simulink model "MicrostickII_ExternalMode"  (R2017b)
settings: Solver=FixedStepDiscrete  StartTime=0.0  StopTime=inf  FixedStep=0.01  RelTol=1e-3
undefined symbols (not defined in the file): A4, B0, B10, B11, B12, Max, MaxPer, ms, P20, P32, P42, P43, Pin, Resol, s, us
libraries: MCHP_Blockset x10
settings Model: SimulationMode=external  ExtModeTrigDuration=1  Creator=M17129  LastModifiedBy=m17129
settings OptimizationCC: PassReuseOutputArgsAs=Individual arguments
settings DebuggingCC: ParameterTunabilityLossMsg=error
settings HardwareCC: ProdBitPerInt=16  ProdBitPerPointer=16  ProdBitPerSizeT=16  ProdBitPerPtrDiffT=16  ProdLargestAtomicInteger=Integer  ProdLargestAtomicFloat=None  ProdWordSize=16  ProdHWDeviceType=Generic->Custom
settings ModelReferenceCC: ModelReferenceNumInstancesAllowed=Single
settings SFSimCC: MATLABDynamicMemAlloc=off
settings RTWCC: SystemTargetFile=MCHP_dsPIC_stf.tlc  TemplateMakefile=MCHP_dsPIC.tmf  Description=Microchip Embedded Target PIC24 dsPIC30 dsPIC33 (real-time)  GenerateReport=on  IncludeHyperlinkInReport=on  LaunchReport=on  CodeExecutionProfiling=on  CodeProfilingInstrumentation=on  GenerateTraceInfo=on  GenerateTraceReport=on  GenerateTraceReportSl=on  GenerateTraceReportSf=on  GenerateTraceReportEml=on  GenerateWebview=on  GenerateCodeMetricsReport=on  GenerateCodeReplacementReport=on
settings CodeAppCC: ForceParamTrailComments=on  IgnoreCustomStorageClasses=off  MaxIdLength=255  OperatorAnnotations=on  SimulinkDataObjDesc=on  SFDataObjDesc=on  InsertBlockDesc=on
settings STFCustomTargetCC: TargetLibSuffix=_lib.a  CodeReplacementLibrary=Microchip® Code Replacement Library for dsPIC  MultiwordLength=256  IncludeMdlTerminateFcn=off  CombineOutputUpdateFcns=on  CombineSignalStateStructs=on  ERTCustomFileBanners=on  SupportContinuousTime=off  RemoveResetFunc=on  MATLABClassNameForMDSCustomization=Simulink.SoftwareTarget.ERTCustomization  GRTInterface=off  SystemTargetFile=MCHP_dsPIC_stf.tlc
settings ERTTargetCC: TargetLibSuffix=_lib.a  CodeReplacementLibrary=Microchip® Code Replacement Library for dsPIC  ParMdlRefBuildCompliant=off  CompOptLevelCompliant=off  ConcurrentExecutionCompliant=off  IncludeMdlTerminateFcn=off  CombineSignalStateStructs=on  SupportNonInlinedSFcns=on  ModelStepFunctionPrototypeControlCompliant=off  CPPClassGenCompliant=off  UseToolchainInfoCompliant=off  ExtMode=on  ExtModeStaticAlloc=on  ExtModeStaticAllocSize=9000  ExtModeMexFile=ext_serial_win32_comm_no_acks  ExtModeMexArgs=1 5 460800  ERTSrcFileBannerTemplate=MCHP_dsPIC_code_template.cgt  ERTHdrFileBannerTemplate=MCHP_dsPIC_code_template.cgt  ERTDataSrcFileTemplate=MCHP_dsPIC_code_template.cgt  ERTDataHdrFileTemplate=MCHP_dsPIC_code_template.cgt  ERTCustomFileTemplate=MCHP_main.tlc

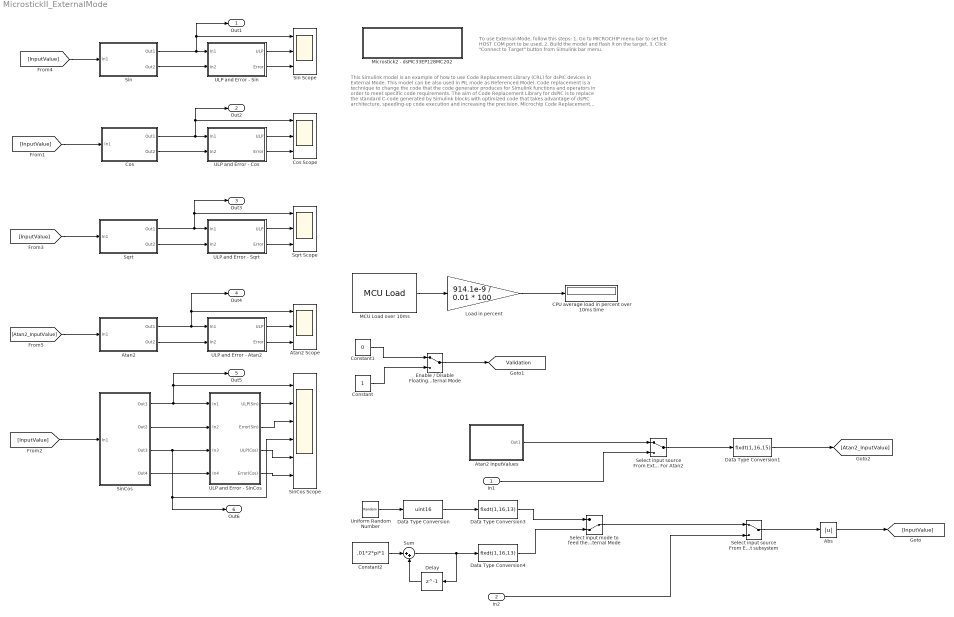
== system MicrostickII_ExternalMode ==
  note: This Simulink model is an example of how to use Code Replacement Library (CRL) for dsPIC devices in External Mode. This model can be also used in PIL mode as Referenced Model.
      |
      | Code replacement is a technique to change the code that the code generator produces for Simulink functions and operators
      | in order to meet specific code requirements. The aim of Code Replacement Library for dsPIC is to replace the standard C-code generated
      | by Simulink blocks with optimized code that takes advantage of dsPIC architecture, speeding-up code execution and increasing the precision.
      |
      | Microchip Code Replacement Library for dsPIC provides support for:
      | - Fixed-Point Matrix Multiplication operations
      | - Fixed-Point Atan2
      | - Fixed-Point Sqrt and Sqrt32
      | - Fixed-Point Sin
      | - Fixed-Point Cos
      | - Fixed-Point SinCos
      | - Abs (absolute value)
      | - Addition and Subtraction with Saturation
      | - Saturation and Cast operations
      |
      | The user can enable Code Replacement Library in two easy steps:
      | 1. Open Configuration Parameters of the Simulink Model
      | 2. From Code Generation --> Interface pane select "Microchip® Code Replacement Library for dsPIC".
      |
      | *You can check which blocks triggered the code replacement by inspecting Code Replacement Report displayed at the end of the build process.
      | *Since this model runs in External Mode you can change the values of tunable parameters (ex. input values for trigonometric functions).
  note: To use External-Mode, follow this steps:
      | 1. Go to MICROCHIP menu bar to set the HOST COM port to be used.
      | 2. Build the model and flash it on the target.
      | 3. Click "Connect to Target" button from Simulink bar menu.
  In1 : Inport  PortDimensions=2
  In2 : Inport  Port=2
  Abs : Abs
  Atan2 : Subsystem
  Atan2 InputValues : Subsystem
  Atan2 Scope : Scope  NumInputPorts=3
  CPU average load in percent over 10ms time : Display
  Constant : Constant  OutDataTypeStr=uint16
  Constant1 : Constant  Value=0  OutDataTypeStr=uint16
  Constant2 : Constant  Value=.01*2*pi*1  OutDataTypeStr=fixdt(1,16,2*pi/65536,0)  SampleTime=.01
  Cos : Subsystem
  Cos Scope : Scope  NumInputPorts=3
  Data Type Conversion : DataTypeConversion  OutDataTypeStr=uint16  ConvertRealWorld=Stored Integer (SI)
  Data Type Conversion1 : DataTypeConversion  OutDataTypeStr=fixdt(1,16,15)  ConvertRealWorld=Stored Integer (SI)
  Data Type Conversion3 : DataTypeConversion  OutDataTypeStr=fixdt(1,16,13)  ConvertRealWorld=Stored Integer (SI)
  Data Type Conversion4 : DataTypeConversion  OutDataTypeStr=fixdt(1,16,13)
  Delay : Delay  DelayLength=1  InitialCondition=0
  Enable / Disable Floating-Point Reference Output *Modifiable in External Mode : ManualSwitch
  Load in percent : Gain  Gain=914.1e-9 / 0.01 * 100  ParamDataTypeStr=Inherit: Inherit from 'Gain'  OutMin=[0]  OutMax=[20]  OutDataTypeStr=single
  MCU Load over 10ms : MCHP_Blockset/Profiling/MCU Load  MCULoadPin=Dynamic Options  MCULoadPin_TXT=None  MCULoadMeasure=on  TIMER_Resolution=Dynamic Options  TIMER_Resolution_TXT="Resol: 0.9143(us)  -  Max: 59.9(ms)"  MCHP_TIMER_REQUEST={MCU_Load}{MCU_Load}21:5:0:0:[]:4194304;  MCHP_TIMER_RESULT=[2 65535 ]  MCHP_MASTERLINK=MicrostickII_ExternalMode/Microstick2 - dsPIC33EP128MC202/Microchip Master  MCHP_COMPILED_INFO="CompiledSampleTime= [0.010000000000000000208   0 ];CompiledInportDataTypes=[ ];CompiledInportDataWidth=[];"  Info="Timer 2:  Resol: 914.0898379(ns)  -  Max: 59.9058(ms)"  SampleTime=0.01
      settings: SourceProductName=MPLAB® Device Blocks for Simulink®
  Microstick2 - dsPIC33EP128MC202 : Subsystem
  Select input mode to feed the functions under test *Modifiable in External Mode : ManualSwitch  CurrentSetting=0
  Select input source From External (input port) / From Current subsystem : ManualSwitch
  Select input source From External (input port) / From Current subsystem For Atan2 : ManualSwitch
  Sin : Subsystem
  Sin Scope : Scope  NumInputPorts=3
  SinCos : Subsystem
  SinCos Scope : Scope  NumInputPorts=6
  Sqrt : Subsystem
  "Sqrt Scope " : Scope  NumInputPorts=3
  Sum : Sum  Inputs=|++  OutDataTypeStr=Inherit: Same as first input
  ULP and Error - Atan2 : Subsystem
  ULP and Error - Cos : Subsystem
  ULP and Error - Sin : Subsystem
  ULP and Error - SinCos : Subsystem
  ULP and Error - Sqrt : Subsystem
  Uniform Random Number : UniformRandomNumber  Minimum=0  Maximum=2^16-1  SampleTime=.01
  Out1 : Outport
  Out2 : Outport  Port=2
  Out3 : Outport  Port=3
  Out4 : Outport  Port=4
  Out5 : Outport  Port=5
  Out6 : Outport  Port=6
  tag scope: Validation=global
  wires:
  [InputValue] -> Sin/1(In1)
  [InputValue] -> Cos/1(In1)
  Select input source From External (input port) / From Current subsystem/1 -> Abs/1
  In2/1 -> Select input source From External (input port) / From Current subsystem/2
  Data Type Conversion3/1 -> Select input mode to feed the functions under test *Modifiable in External Mode/1
  ULP and Error - Sqrt/2(Error) -> "Sqrt Scope "/3
  Cos/1(Out1) -> Cos Scope/1, Out2/1, ULP and Error - Cos/1(In1)
  SinCos/1(Out1) -> Out5/1, SinCos Scope/1, ULP and Error - SinCos/1(In1)
  Cos/2(Out2) -> ULP and Error - Cos/2(In2)
  Constant1/1 -> Enable / Disable Floating-Point Reference Output *Modifiable in External Mode/1
  SinCos/4(Out4) -> ULP and Error - SinCos/4(In4)
  Atan2/1(Out1) -> Atan2 Scope/1, Out4/1, ULP and Error - Atan2/1(In1)
  ULP and Error - Cos/2(Error) -> Cos Scope/3
  ULP and Error - SinCos/3(ULP(Cos)) -> SinCos Scope/5
  ULP and Error - Atan2/1(ULP) -> Atan2 Scope/2
  Delay/1 -> Sum/2
  ULP and Error - Sqrt/1(ULP) -> "Sqrt Scope "/2
  Sqrt/1(Out1) -> "Sqrt Scope "/1, Out3/1, ULP and Error - Sqrt/1(In1)
  Data Type Conversion4/1 -> Select input mode to feed the functions under test *Modifiable in External Mode/2
  Data Type Conversion1/1 -> [Atan2_InputValue]
  SinCos/3(Out3) -> SinCos Scope/4, Out6/1, ULP and Error - SinCos/3(In3)
  ULP and Error - SinCos/4(Error(Cos)) -> SinCos Scope/6
  Sin/2(Out2) -> ULP and Error - Sin/2(In2)
  ULP and Error - Atan2/2(Error) -> Atan2 Scope/3
  ULP and Error - Cos/1(ULP) -> Cos Scope/2
  Data Type Conversion/1 -> Data Type Conversion3/1
  Sqrt/2(Out2) -> ULP and Error - Sqrt/2(In2)
  SinCos/2(Out2) -> ULP and Error - SinCos/2(In2)
  ULP and Error - Sin/1(ULP) -> Sin Scope/2
  MCU Load over 10ms/1 -> Load in percent/1
  Constant2/1 -> Sum/1
  Atan2/2(Out2) -> ULP and Error - Atan2/2(In2)
  Sum/1 -> Data Type Conversion4/1, Delay/1
  Sin/1(Out1) -> Out1/1, Sin Scope/1, ULP and Error - Sin/1(In1)
  [InputValue] -> Sqrt/1(In1)
  Uniform Random Number/1 -> Data Type Conversion/1
  ULP and Error - SinCos/1(ULP(Sin)) -> SinCos Scope/2
  Enable / Disable Floating-Point Reference Output *Modifiable in External Mode/1 -> [Validation]
  Constant/1 -> Enable / Disable Floating-Point Reference Output *Modifiable in External Mode/2
  ULP and Error - Sin/2(Error) -> Sin Scope/3
  In1/1 -> Select input source From External (input port) / From Current subsystem For Atan2/2
  [InputValue] -> SinCos/1(In1)
  Abs/1 -> [InputValue]
  Select input mode to feed the functions under test *Modifiable in External Mode/1 -> Select input source From External (input port) / From Current subsystem/1
  Select input source From External (input port) / From Current subsystem For Atan2/1 -> Data Type Conversion1/1
  [Atan2_InputValue] -> Atan2/1(In1)
  Atan2 InputValues/1(Out1) -> Select input source From External (input port) / From Current subsystem For Atan2/1
  ULP and Error - SinCos/2(Error(Sin)) -> SinCos Scope/3
  Load in percent/1 -> CPU average load in percent over 10ms time/1

== system MicrostickII_ExternalMode/Atan2 ==
  In1 : Inport
  Atan2 Q15 : Subsystem
  Double Atan2 - Reference : Subsystem  TreatAsAtomicUnit=on
  Out1 : Outport
  Out2 : Outport  Port=2
  wires:
  In1/1 -> Atan2 Q15/1(In1), Double Atan2 - Reference/1(In1)
  Double Atan2 - Reference/1(Simulink_Out_Q1.15) -> Out2/1
  Atan2 Q15/1(Out1) -> Out1/1
  [Validation] -> Double Atan2 - Reference/Enable

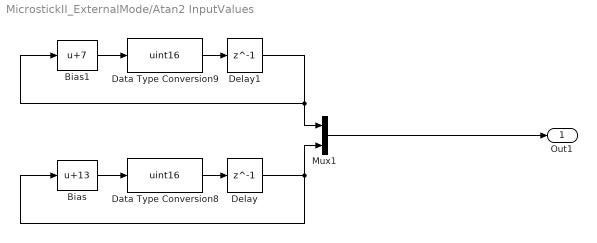
== system MicrostickII_ExternalMode/Atan2 InputValues ==
  Bias : Bias  Bias=13
  Bias1 : Bias  Bias=7
  Data Type Conversion8 : DataTypeConversion  OutDataTypeStr=uint16  ConvertRealWorld=Stored Integer (SI)
  Data Type Conversion9 : DataTypeConversion  OutDataTypeStr=uint16  ConvertRealWorld=Stored Integer (SI)
  Delay : Delay  DelayLength=1  InitialCondition=0
  Delay1 : Delay  DelayLength=1  InitialCondition=0
  Mux1 : Mux  Inputs=2
  Out1 : Outport
  wires:
  Delay/1 -> Bias/1, Mux1/2
  Data Type Conversion8/1 -> Delay/1
  Delay1/1 -> Mux1/1, Bias1/1
  Bias1/1 -> Data Type Conversion9/1
  Data Type Conversion9/1 -> Delay1/1
  Mux1/1 -> Out1/1
  Bias/1 -> Data Type Conversion8/1

== system MicrostickII_ExternalMode/Cos ==
  In1 : Inport
  Cos Double - Reference : Subsystem
  Cos Q15 : Subsystem
  Out1 : Outport
  Out2 : Outport  Port=2
  wires:
  In1/1 -> Cos Q15/1(In2), Cos Double - Reference/1(In1)
  Cos Double - Reference/1(Out1) -> Out2/1
  Cos Q15/1(Cos_Out1) -> Out1/1
  [Validation] -> Cos Double - Reference/Enable

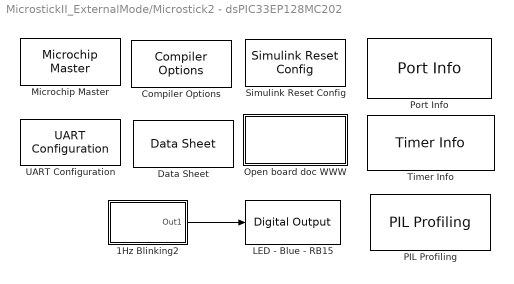
== system MicrostickII_ExternalMode/Microstick2 - dsPIC33EP128MC202 ==
  1Hz Blinking2 : Subsystem
  Compiler Options : MCHP_Blockset/System Configuration/Compiler Options  Priority=1  LATEST_CMPLR=on  COMP_LIST=Dynamic Options  COMP_LIST_TXT=xc16 - v1.33  USE_64BIT_DOUBLE=off  MCHP_MULTITHREAD_COMPILATION=on  UseCustom_LinkerScript=off  MCHP_MASTERLINK=MicrostickII_ExternalMode/Microstick2 - dsPIC33EP128MC202/Microchip Master  OPTIMIZATION_LEVEL=3  MPLAB_LINKLIB=default  MPLAB_LINKLIB1=default  UNROLL_LOOPS=on  OMIT_FRAME_POINTER=off  PROCEDURAL_ABSTRACTION=off  MCONST=in data memory  MDATA=Use only memory below address 8192 (faster)  MSCALAR=Use only memory below address 8192 (faster)  MCODE=is less than 32768 (faster)  HEAP_SIZE=0  OMF=elf  DEBUG_INFO=off  AssemblyListing=off  ProduceHexOutput=on
      settings: SourceProductName=MPLAB® Device Blocks for Simulink®
  Data Sheet : MCHP_Blockset/System Info/Data Sheet  DOC_Type=datasheet  DOC_MCHP_Id=33FJ64MC802  DOC_FileLastCheckTime=[0 0 0 0 0 0]  cpy_MCHP_Id=33EP128MC202  MCHP_MASTERLINK=MicrostickII_ExternalMode/Microstick2 - dsPIC33EP128MC202/Microchip Master
      settings: AttributesFormatString=%<cpy_MCHP_Id>  SourceProductName=MPLAB® Device Blocks for Simulink®
  LED - Blue - RB15 : MCHP_Blockset/Digital IO/Digital Output  PORT=Dynamic Options  PORT_TXT="B   [ 0 : 15 ]"  PIN=[13]  PACK=off  SIMULTANEOUS=off  READPREVIOUS=off  ORDERING=None  SampleTime=-1  MCHP_MASTERLINK=MicrostickII_ExternalMode/Microstick2 - dsPIC33EP128MC202/Microchip Master
      settings: SourceProductName=MPLAB® Device Blocks for Simulink®
  Microchip Master : MCHP_Blockset/System Configuration/Microchip Master  Priority=1  PICREF=33EP128MC202  TIMESTEP_REF="Timer  ( 0.01s + [0.0014283%] ==> 0.01s )"  BUSYFLAG=Dynamic Options  BUSYFLAG_TXT=B12 / Pin[23]  PWRTEN=Not used  BOREN=Disable  BODENV=2.7V  BORV=Not used  FPWRT=128ms  DSBOREN=Enable ZPBOR during Deep Sleep Mode  DSLPBOR=Not used  MCLRE=Enabled  SMCLR=MCLR pin generates a normal system Reset  PMDL1WAY=Allow only one reconfiguration  RSTPRI=Device will obtain reset instruction from Primary flash  TEMP=Not used  SOSCSRC=Not used  SOSCSEL=Not used  IOL1WAY=Allow only one reconfiguration  ALTVREF=Not used  DISUVREG=Not used  DSSWEN=Not used  LPCFG=Not used  RTCBAT=Not used  VBTBOR=Not used  WUTSEL=Not used  POWERSAVE=off  FNOSC=Internal Fast RC (FRC)  FPR=ECIO w/ PLL 16x  FOSFPR=HS3 w/PLL 16x  FOS=Primary Oscillator  FRANGE=High Range  OSCILLATOR_SELECT=Internal Fast RC (FRC)  OSCILLATOR_SELECT_spd=Internal Fast RC (FRC)  QUARTZ=7.37e+06  QUARTZ_spd=7.37e+06  POSCGAIN=2x gain setting  POSCBOOST=Boost the kick start of the oscillator  SOSCGAIN=2x gain setting  SOSCBOOST=Boost the kick start of the oscillator  ACTIV_PLL=on  ACTIV_PLL_spd=on  MIPS_DESIRED=70e+06  MIPS_DESIRED_spd=70e+06  FPLLMUL=Not used  FPLLIDIV=8x Divider  POSCFREQ=Not used  POSCMD=Primary Oscillator Disabled  POSCMOD=Primary osc disabled  MIPS=70.01500000000000056843419 * 1e6  ACLKCON=Optimized for PWM resolution & ADC conversion speed  FPLLODIV=32x Divider  PLLKEN=Clock switch to PLL source will wait until the PLL lock signal is valid.  FCKSM=Clock switching is enabled;Fail-safe Clock Monitor is disabled  FCKSMEN=Sw Disabled; Mon Disabled  IESO=Start up with FRC; then switch  DSWDTPS=1:2^36  FWDTEN=Disable  FWDTWINSZ=Window size is 25%  FWPSA=1:512  FWPSA0=1:128  FWPSB=1:16  WDT=Disable  WDTPOST=1:32768  WDTPRE=1:128  WDTPS=1:1048576  WINDIS=Watchdog Timer in Non-Window mode  WWDTEN=Non-Window mode  DSWDTEN=Enable DSWDT during Deep Sleep Mode  DSWDTOSC=Select LPRC as DSWDT Reference clock  FPBDIV=Not used  FSOSCEN=Enable SOSC  LPRCSEL=Not used  OSCIOFCN=Not used  OSCIOFNC=OSC2 is general purpose digital I/O pin  LVRCFG=Not used  PLL_96MHZ=Not used  PLL96MHZ=Not used  PLLDIV=Not used  WDTCLK=Not used  WDTCMX=Not used  WDTWIN=WDT Window is 25% of WDT period  APL=Aux Flash Code protect is disabled  APLK=Aux Flash Write Protection and Code Protection is Disabled  AWRP=Auxiliary program memory is not write-protected  BSS=No Boot program Flash segment  BWP=Not used  BWRP=Boot Segment may be written  CP=Protection Disabled  EBS=No Boot EEPROM  ESS=No Segment Data EEPROM  GCP=General Segment Code protect is Disabled  GSS=General Segment Code protect is Disabled  GSS0=Not used  GSSK=General Segment Write Protection and Code Protection is Disabled  GWRP=General Segment may be written  PWP=Not used  RBS=No Boot RAM  RSS=No Secure RAM  SSS=No Secure Segment  SWRP=Secure segment may be written  WPCFG=Not used  WPDIS=Not used  WPEND=Not used  WPFP=Not used  ICESEL=Communicate on PGEC1/PGED1  ICS=Communicate on PGEC1 and PGED1  JTAGEN=Disable  COE=Not used  RES=Not used  DEBUG=Debugger is disabled  BACKBUG=Not used  BKBUG=Not used  ALTI2C=I2C mapped to SDA1/SCL1 pins  ALTI2C1=I2C1 mapped to SDA1/SCL1 pins  ALTI2C2=I2C2 mapped to SDA2/SCL2 pins  ALTQIO=QEA1; QEB1; INDX1 are selected as inputs to QEI1  ALTSS1=SS1A is selected as the I/O pin for SPI1  CMPPOL0=Hysteresis is applied to falling edge  CMPPOL1=Hysteresis is applied to falling edge  FCANIO=Not used  FETHIO=Default Ethernet I/O  FMIIEN=MII Enabled  FSRSSEL=Not used  FUSBIDIO=Controlled by the USB Module  FVBUSONIO=Not used  HPOL=PWM module high side output pins have active-high output polarity  HYST0=45 mV Hysteresis  HYST1=45 mV Hysteresis  I2C1SEL=Not used  LPOL=PWM module low side output pins have active-high output polarity  PWMPIN=PWM module pins controlled by PORT register at device Reset  RTCOSC=Not used  UPLLEN=USB PLL is enabled  UPLLIDIV=Not used  ATMOD8=Not used  ALTPMP=Not used  I2C2SEL=Not used  ALTADREF=Not used  ALTCVREF=Not used  PWMLOCK=PWM registers may be written without key sequence  MCHP_TIMER_REQUEST={Time Step}{TS}0:2:3:1:[]:700150;  MCHP_TIMER_RESULT=[1 10938.843749999992724 ]  MCHP_PORT={Busy Flag}{Busy}0:1:B12;  MCHP_PLLRegisters="[5    264  16387     -1]"  MCHPVAR=MCHP.fcy.MIPS=70015000;MCHP.fcy.SYSCLK=70015000;MCHP.fcy.ADC=70015000;MCHP.fcy.Comparator=70015000;MCHP.fcy.I2C=70015000;MCHP.fcy.SPI=70015000;MCHP.fcy.UART=70015000;MCHP.fcy.Timers=70015000;MCHP.fcy.OC=70015000;MCHP.fcy.IC=70015000;MCHP.fcy.Ports=70015000;MCHP.fcy.QEI=70015000;MCHP.PowerSave=0;MCHP.TimeStepFactor=MCHP_Fun.Hex2num('[3FF0000EF9F87D69]');MCHP.TimeStep_Timer=1;MCHP.NTIMERS=5;MCHP.id.name='33EP128MC202';MCHP.id.N=reshape([33 128 202],1,3);MCHP.id.L=reshape({ 'EP','MC',''},1,3);MCHP.id.Arch=3;MCHP.periph.PPS.reg_RPINRx=reshape([-1 1 1 -1 -1 -1 1 -1 -1 -1 -1 -1 -1 -1 1 1 1 1 -1 -1 -1 -1 -1 -1 1 1 -1 -1 1 1 1 1 -1 -1 -1 -1 1 -1 1 -1 -1 -1 -1 -1 1 1 1 -1 -1 -1 -1 -1 1 -1 -1 -1 -1 -1 -1 -1 -1 -1 -1 -1 -1 -1 -1 -1 -1 -1 -1 -1 -1 -1 -1 1 -1 1 1 1],1,80);MCHP.PPS.dsPIC.RP=reshape([-1 -1 -1 -1 -1 -1 -1 -1 -1 -1 -1 -1 -1 -1 -1 -1 -1 -1 -1 -1 4 -1 -1 -1 -1 -1 -1 -1 -1 -1 -1 -1 -1 -1 -1 19 20 21 22 23 24 25 26 27],1,44);MCHP.PPS.dsPIC.RPI=reshape([-1 -1 -1 -1 -1 -1 -1 -1 -1 -1 -1 -1 -1 -1 -1 -1 -1 -1 -1 -1 -1 -1 -1 -1 -1 -1 -1 -1 -1 -1 -1 -1 16 17 18 -1 -1 -1 -1 -1 -1 -1 -1 -1 28 29 30 31],1,48);MCHP.PPS.dsPIC.RPINR_list=reshape({ '1','INT1','INT2','INT3','INT4','T1CK','T2CK','T3CK','T4CK','T5CK','T6CK','T7CK','T8CK','T9CK','IC1','IC2','IC3','IC4','IC5','IC6','IC7','IC8','OCFA','OCFB','FLT1','FLT2','FLT3','FLT4','QEA1','QEB1','INDX1','HOME1','QEA2','QEB2','INDX2','HOME2','U1RX','U1CTS','U2RX','U2CTS','SDI1','SCK1_in','SS1_in','44','SDI2','SCK2_in','SS2_in','48','CSDIR','CSCK','COFS','52','C1RX','C2RX','U3RX','U3CTS','U4RX','U4CTS','SDI3','SCK3_in','SS3_in','62','SDI4','SCK4_in','SS4_in','66','IC9','IC10','IC11','IC12','IC13','IC14','IC15','IC16','OCFC','SYNCI1','SYNCI2','DTCMP1','DTCMP2','DTCMP3','DTCMP4','DTCMP5','DTCMP6','DTCMP7','FLT5','FLT6','FLT7','FLT8','89','SENT1','SENT2','92'},1,92);MCHP.PPS.dsPIC.RPOR_list=reshape({ '1','U1TX','U1RTS','U2TX','U2RTS','SDO1','SCK1_out','SS1_out','SDO2','SCK2_out','SS2_out','CSDO','CSCK','COFS','C1TX','C2TX','OC1','OC2','OC3','OC4','OC5','OC6','OC7','OC8','C1OUT','C2OUT','C3OUT','U3TX','U3RTS','U4TX','U4RTS','SDO3','SCK3_out','SS3_out','SDO4','SCK4_out','SS4_out','OC9','OC10','OC11','OC12','OC13','OC14','OC15','OC16','SYNCO1','SYNCO2','QEI1CCMP','QEI2CCMP','REFCLK','C4OUT','C5OUT','52','53','54','55','56','SENT1','SENT2'},1,59);MCHP.PPS.map_RPnR_RPORx=reshape([20 35 36 37 38 39 40 41 42 43],1,10);MCHP.Rx=reshape([2 4 -1 -1 -1 -1 -1 -1 -1 -1 -1 3 5 -1 -1 -1 -1 -1 -1 -1 -1 -1 9 6 -1 -1 -1 -1 -1 -1 -1 -1 -1 10 7 -1 -1 -1 -1 -1 -1 -1 -1 -1 12 11 -1 -1 -1 -1 -1 -1 -1 -1 -1 -1 14 -1 -1 -1 -1 -1 -1 -1 -1 -1 -1 15 -1 -1 -1 -1 -1 -1 -1 -1 -1 -1 16 -1 -1 -1 -1 -1 -1 -1 -1 -1 -1 17 -1 -1 -1 -1 -1 -1 -1 -1 -1 -1 18 -1 -1 -1 -1 -1 -1 -1 -1 -1 -1 21 -1 -1 -1 -1 -1 -1 -1 -1 -1 -1 22 -1 -1 -1 -1 -1 -1 -1 -1 -1 -1 23 -1 -1 -1 -1 -1 -1 -1 -1 -1 -1 24 -1 -1 -1 -1 -1 -1 -1 -1 -1 -1 25 -1 -1 -1 -1 -1 -1 -1 -1 -1 -1 26 -1 -1 -1 -1 -1 -1 -1 -1 -1],11,16);MCHP.ADC.ANtype=reshape([3 0],1,2);MCHP.ADC.ADCONx=reshape([47103 59391 40959 263 0 0],1,6);MCHP.ADC.ADCHS_0=reshape([40863 1799],1,2);MCHP.ADC.Flags=reshape([1 0],1,2);MCHP.ADC.Buffer=reshape([16 -1],1,2);MCHP.ADC.port=reshape([0 1 16 17 18 19 -1 -1 -1 -1 -1 -1 -1 -1 -1 -1 -1 -1 -1 -1 -1 -1 -1 -1 -1 -1 -1 -1 -1 -1 -1 -1 -1 -1 -1 -1 -1 -1 -1 -1 -1 -1 -1 -1 -1 -1 -1 -1 -1 -1 -1 -1 -1 -1 -1 -1 -1],1,57);MCHP.ADC.port_ALT=reshape([-1 -1 -1 -1],1,4);MCHP.ADC.port_VrefP=17;MCHP.ADC.port_VrefM=16;MCHP.ADC.port_AVdd=-1;MCHP.ADC.port_AVss=-1;MCHP.ADC.ADCDATA=reshape([0 0 0 0 0 0 0 0 0 0 0 0 0 0 0 0 0 0 0 0 0 0 0 0 0 0 0 0 0 0 0 0 0 0 0 0 0 0 0 0 0 0 0 0 0 0 0 0 0 0 0 0 0 0 0 0 0],1,57);MCHP.memory.RAM=16384;MCHP.memory.RAM_XBegin=4096;MCHP.memory.RAM_YBegin=12288;MCHP.memory.RAM_dma=reshape([-1 -1],1,2);MCHP.memory.FLASH_ECC=0;MCHP.DMA.Num=4;MCHP.DMA.CNTmax=16383;MCHP.QEI.QEICONx=reshape([49023 -1 -1 -1 -1 -1],1,6);MCHP.QEI.QEItype=1;MCHP.QEI.Port_QEI_INDX=reshape([-1 -1],1,2);MCHP.QEI.Port_QEI_QEA=reshape([-1 -1],1,2);MCHP.QEI.Port_QEI_QEB=reshape([-1 -1],1,2);MCHP.QEI.Port_QEI_UPDN=reshape([-1 -1],1,2);MCHP.INT.Port=reshape([23 32767 32767 -1 -1],1,5);MCHP.PWM_HS.Flags=reshape([3 1 0],1,3);MCHP.PWM.port_FLT=reshape([-1 -1 -1 -1 -1 -1 -1 -1 -1 -1 -1 -1 -1 -1 -1 -1 -1 -1 -1 -1 -1 -1 -1 -1 -1 -1 -1 -1 -1 -1 -1 -1 20],1,33);MCHP.PWM.PWMRef=-1;MCHP.PWM.Flag=0;MCHP.PWM.Port_PWM_l=reshape([31 -1 29 -1 27 -1 -1 -1 -1 -1 -1 -1 -1 -1 -1 -1 -1 -1 -1 -1 -1 -1 -1 -1],2,12);MCHP.PWM.Port_PWM_h=reshape([30 -1 28 -1 26 -1 -1 -1 -1 -1 -1 -1 -1 -1 -1 -1 -1 -1 -1 -1 -1 -1 -1 -1],2,12);MCHP.IC.Port=reshape([32767 32767 32767 32767 0 0 0 0 0 0 0 0 0 0 0 0],1,16);MCHP.IC.type=1;MCHP.OC.Port=reshape([32767 32767 32767 32767 0 0 0 0 0 0 0 0 0 0 0 0],1,16);MCHP.OC.type=1;MCHP.CN.Port=reshape([-1 -1 -1 -1 -1 -1 -1 -1 -1 -1 -1 -1 -1 -1 -1 -1 -1 -1 -1 -1 -1 -1 -1 -1 -1 -1 -1 -1 -1 -1 -1 -1 -1 -1 -1 -1 -1 -1 -1 -1 -1 -1 -1 -1 -1 -1 -1 -1 -1 -1 -1 -1 -1 -1 -1 -1 -1 -1 -1 -1 -1 -1 -1 -1 -1 -1 -1 -1 -1 -1 -1 -1 -1 -1 -1 -1 -1 -1 -1 -1 -1 -1 -1 -1 -1],1,85);MCHP.CN.PullUp=reshape([31 65535 0 0 0 0 0 0 0 0 0],1,11);MCHP.CN.type=1;MCHP.CN.Flag_PullDown=1;MCHP.SPI.Refs=reshape([1 2 0 0 0 0],1,6);MCHP.SPI.SPIxCON1=8191;MCHP.SPI.SPIxCON2=57347;MCHP.SPI.Port_SDI=reshape([25 -1 -1 -1 -1 -1],1,6);MCHP.SPI.Port_SDO=reshape([24 -1 -1 -1 -1 -1],1,6);MCHP.SPI.Port_SCK=reshape([23 -1 -1 -1 -1 -1],1,6);MCHP.SPI.Port_SS=reshape([16 -1 -1 -1 -1 -1],1,6);MCHP.I2C.Refs=reshape([1 2 0 0 0],1,5);MCHP.I2C.I2CxCON=49151;MCHP.I2C.NewRegName=1;MCHP.I2C.Port_SDA=reshape([-1 -1 -1 -1 -1],1,5);MCHP.I2C.Port_SCL=reshape([-1 -1 -1 -1 -1],1,5);MCHP.I2C.Port_ASDA=reshape([25 21 -1 -1 -1],1,5);MCHP.I2C.Port_ASCL=reshape([24 22 -1 -1 -1],1,5);MCHP.I2C.Fuse_Port_SCL_SDA=reshape([3 1 4 1 -1 -1 -1 -1 -1 -1],2,5);MCHP.I2C.Fuse_Port_ASCL_ASDA=reshape([3 2 4 2 -1 -1 -1 -1 -1 -1],2,5);MCHP.Comp.Port_CVrefin=-1;MCHP.Comp.Port_CVref=-1;MCHP.Comp.Port_CVref1O=24;MCHP.Comp.Port_CVref2O=4;MCHP.Comp.Port_CxOUT=reshape([32767 32767 32767 32767 -1],1,5);MCHP.Comp.Port_OAxOUT=reshape([17 0 -1 -1 -1],1,5);MCHP.Comp.Port_CxINP=reshape([18 1 -1 -1 -1],1,5);MCHP.Comp.Port_CxINM=reshape([19 -1 -1 -1 16 -1 -1 -1 -1 -1 -1 -1 -1 -1 -1 -1 -1 -1 -1 -1],4,5);MCHP.Comp.nComp=reshape([4 0 0],1,3);MCHP.Comp.OpAmp=3;MCHP.Comp.CVRCON=reshape([17663 0],1,2);MCHP.CDAC.Port_DACx=reshape([-1 -1 -1],1,3);MCHP.CDAC.nCDAC=0;MCHP.UART.port_Rx=reshape([32767 32767 -1 -1 -1 -1],1,6);MCHP.UART.port_Tx=reshape([32767 32767 -1 -1 -1 -1],1,6);MCHP.UART.port_ARx=reshape([-1 -1],1,2);MCHP.UART.port_ATx=reshape([-1 -1],1,2);MCHP.UART.port_RTS=reshape([32767 32767 -1 -1 -1 -1],1,6);MCHP.UART.port_CTS=reshape([32767 32767 -1 -1 -1 -1],1,6);MCHP.UART.reg_UxMODE=reshape([48127 48127 -1 -1 -1 -1],1,6);MCHP.UART.reg_UxSTA=reshape([61439 61439 -1 -1 -1 -1],1,6);MCHP.modsrc.DOS_00794=1;MCHP.modsrc.DOS_00931=1;MCHP.modsrc.DOS_00932=1;MCHP.modsrc.DOS_00942=1;MCHP.modsrc.DOS_00938=1;MCHP.modsrc.DOS_00996=1;MCHP.modsrc.DOS_00997=1;MCHP.modsrc.DOS_00998=1;MCHP.modsrc.DOS_00209=0;MCHP.modsrc.DOS_01555_adc=0;MCHP.modsrc.DOS_01293=1;MCHP.modsrc.DOS_00828=0;MCHP.modsrc.DOS_01116=1;MCHP.modsrc.DOS_01017_RPORx=1;MCHP.modsrc.DOS_01017_RPINRx=1;MCHP.modsrc.DOS_01555_nvm_tsmc18_v2_16bit=0;MCHP.modsrc.DOS_00804=1;MCHP.modsrc.DOS_00826=1;MCHP.modsrc.DOS_01555_TLAK_PMDx=0;MCHP.modsrc.DOS_01555_TLAK_INT_=0;MCHP.modsrc.DOS_00933=1;MCHP.modsrc.DOS_01555=0;MCHP.modsrc.DOS_01555_ptg=0;MCHP.modsrc.DOS_00929=1;MCHP.modsrc.DOS_00958=1;MCHP.modsrc.DOS_01117_PORTx=1;MCHP.modsrc.DOS_00999=0;MCHP.modsrc.DOS_01198=0;MCHP.modsrc.DOS_01041=1;MCHP.modsrc.DOS_00892=1;MCHP.modsrc.DOS_01287_TLAC_PMDx=1;MCHP.modsrc.DOS_01287_TLAC_INT_=1;MCHP.modsrc.DOS_01424=1;MCHP.modsrc.DOS_01332=1;MCHP.modsrc.DOS_01441_i2c_upb_v1_16bit_TLAH=0;MCHP.modsrc.DOS_01482=0;MCHP.modsrc.DOS_02508c11=0;MCHP.modsrc.DOS_01468_PMBA_current_source=0;MCHP.modsrc.DOS_02291_PGA=0;MCHP.modsrc.DOS_01467_Comparator=0;MCHP.modsrc.DOS_01498_TLAY=0;MCHP.modsrc.DOS_02316_nvm_ctrl_v1_16bit=0;MCHP.modsrc.DOS_00993_PLL_120MHz=0;MCHP.modsrc.DOS_01577_cla_clc_upb_v1=0;MCHP.modsrc.DOS_01332_ptg_pc_v1=0;MCHP.modsrc.DOS_00958_pwm_TLAY=0;MCHP.modsrc.TLAY_IOPorts=0;MCHP.modsrc.DOS_00929q=0;MCHP.modsrc.DOS_02415_spi_v5=0;MCHP.modsrc.DOS_RPINRx_16bit_2=0;MCHP.modsrc.DOS_01497_TLAH_PMDx=0;MCHP.modsrc.DOS_02550_TLAL_INT=0;MCHP.modsrc.DOS_00958_pwm_TLAH=0;MCHP.modsrc.DOS_01287_TLAH_INT_=0;MCHP.modsrc.DOS_01113=0;MCHP.modsrc.DOS_01017_PMDx=0;MCHP.modsrc.DOS_00927=0;MCHP.modsrc.DOS_01080=0;MCHP.modsrc.DOS_00794_cpu_16bit_v3=0;MCHP.modsrc.DOS_02359a_sent_j2716_upb_v1=0;MCHP.modsrc.DOS_01520_wdt_dmt_upb_v1_16bit=0;MCHP.modsrc.DOS_02192_TLCD_PMDx=0;MCHP.modsrc.DOS_02192_TLCD_INT_=0;MCHP.modsrc.DOS_02192_cmp=0;MCHP.modsrc.DOS_00958_pwm_TLCD=0;MCHP.modsrc.DOS_02192_PORTx_TLCD=0;MCHP.modsrc.DOS_00936=0;MCHP.modsrc.DOS_00995=0;MCHP.modsrc.DOS_00546=0;MCHP.modsrc.DOS_00474=0;MCHP.modsrc.DOS_02481_WACJ_Config=0;MCHP.modsrc.DOS_02569_pfm_cache_ocp_v1=0;MCHP.modsrc.DOS_02819_pfm_ctrl_32bit_upb_v2=0;MCHP.modsrc.DOS_02674_wdt_upb_v1_32bit=0;MCHP.modsrc.DOS_01520_wdt_dmt_upb_v1=0;MCHP.modsrc.DOS_02869_icd_jtag_bvci_upb_v2=0;MCHP.modsrc.DOS_02823_WACJ_clk_cru_upb_v2=0;MCHP.modsrc.DOS_01423_RPINRx=0;MCHP.modsrc.DOS_02481_RPORx=0;MCHP.modsrc.DOS_02511_pwr_sib_upb_v1_32bit=0;MCHP.modsrc.DOS_02481_WACJ_int_evic_v3=0;MCHP.modsrc.DOS_01500_dma_bvci_v2=0;MCHP.modsrc.DOS_02141_tmr_classa_pb_v2=0;MCHP.modsrc.DOS_02815_tmr_classb_upb_v1=0;MCHP.modsrc.DOS_00740_icap_pb_v1=0;MCHP.modsrc.DOS_00749_ocmp_pb_v1=0;MCHP.modsrc.DOS_01441_i2c_upb_v1_32bit=0;MCHP.modsrc.DOS_01329_spi_pb_v2=0;MCHP.modsrc.DOS_02478_uart_irda_upb_v1_32bit=0;MCHP.modsrc.DOS_02514_dfm_strl_sst_upb_v1=0;MCHP.modsrc.DOS_01427_cmp_control_upb_v1_32bit=0;MCHP.modsrc.DOS_01445_dac_nbit__control_upb_v1_32bit=0;MCHP.modsrc.DOS_01461_afe_ctmu_con_upb_v1=0;MCHP.modsrc.DOS_02472_ppi_pmp16_upb_v1=0;MCHP.modsrc.DOS_02467_gpio_ports_upb_v1=0;MCHP.modsrc.DOS_02508_adc_sar_ctrl_upb_v1_PIC32MK=0;MCHP.modsrc.DOS_02813a_usb_otgcore_pb_v3=0;MCHP.modsrc.DOS_01261_tmr_rtcc_pb_v2=0;MCHP.modsrc.DOS_01475_lpwr_deep_sleep_ctrl_v2=0;MCHP.modsrc.DOS_EIP_00136_ssx_v1=0;MCHP.modsrc.DOS_01152_can_bvci_v1=0;MCHP.modsrc.DOS_02481_WACN_Config=0;MCHP.modsrc.DOS_02823_WACN_clk_cru_upb_v2=0;MCHP.modsrc.DOS_02481_WACN_int_evic_v3=0;MCHP.modsrc.DOS_03554_cmp_control_upb_v2_32bit=0;MCHP.modsrc.DOS_01577_cla_clc_upb_v1_32bit=0;MCHP.modsrc.DOS_03247_can_fd_upb_v2=0;MCHP.modsrc.DOS_02481_WACK_MC_Config=0;MCHP.modsrc.DOS_03247_can_fd_upb_v2_pic32mk=0;MCHP.modsrc.DOS_02481_WACJ_MC_Config=0;MCHP.modsrc.DOS_02481_WACJ_MC_int_evic_v3=0;MCHP.modsrc.DOS_01477_pwm_mc_upb_v1=0;MCHP.modsrc.DOS_01459_ptg_pc_upb_v1_SIC=0;MCHP.modsrc.DOS_01494_qei_32b_upb_v1=0;MCHP.modsrc.DOS_02481_WACN_MC_Config=0;MCHP.modsrc.DOS_02481_WACN_MC_int_evic_v3=0;MCHP.modsrc.DOS_01599_WAAA_Config=0;MCHP.modsrc.DOS_01549_pfm_control_hpmd_v3=0;MCHP.modsrc.DOS_01385_wdt_pwrt_pb_v2a=0;MCHP.modsrc.DOS_00800_dac_4bit_ctrl_pb_v1=0;MCHP.modsrc.DOS_01539_icd_jtag_pb_v2=0;MCHP.modsrc.DOS_01545_clk_cru_upb_v1=0;MCHP.modsrc.DOS_01423_RPORx=0;MCHP.modsrc.DOS_01522_WAAA_int_evic_v2=0;MCHP.modsrc.DOS_00734_uart_irda_pb_v1=0;MCHP.modsrc.DOS_00751_ppi_pmp_v1=0;MCHP.modsrc.DOS_00687_tmr_classa_pb_v1=0;MCHP.modsrc.DOS_00745_tmr_classb_pb_v1=0;MCHP.modsrc.DOS_01405_adc_pc_ctrl_upb_v1=0;MCHP.modsrc.DOS_00866_cmp_control_pb_v2=0;MCHP.modsrc.DOS_01599_WAAA_Ports=0;MCHP.modsrc.DOS_01114_eth_bvci_v1=0;MCHP.modsrc.DOS_01643_pfm_cache_ahb_v2=0;MCHP.modsrc.DOS_EIP_00123_sqi_v1=0;MCHP.modsrc.DOS_EIP_00124_usb_hs_otgcore_v1=0;MCHP.modsrc.DOS_EIP_00159_math_rng_ahbs_v1=0;MCHP.modsrc.DOS_EIP_00109_ebi_v1=0;MCHP.modsrc.DOS_EIP_00158_crypto_v1=0;MCHP.modsrc.DOS_02787_WACD_Config=0;MCHP.modsrc.DOS_02823_clk_cru_upb_v2=0;MCHP.modsrc.DOS_02907_WACD_int_evic_v3=0;MCHP.modsrc.DOS_02508_adc_sar_ctrl_upb_v1=0;MCHP.modsrc.DOS_02831_usb_clk_rst_v2=0;MCHP.modsrc.DOS_EIP_00206r5_sqi_v2=0;MCHP.modsrc.DOS_EIP_00218_math_rng_ahbs_v2=0;MCHP.clock.PBxDIV=-1;  MCHP_CRC=6327243  BTMODE=Not used  RES1=Not used  PLLSS=Not used  RES2=Not used  ALTCMPI=Not used  BOREN1=Not used  ALTRB6=Not used  RETCFG=Not used  DFMCY=Not used  BSS2=No Boot Segment  BSEN=No Boot Segment  CWRP=Configuration Segment may be written  CSS=No Protection (other than CWRP)  AIVTDIS=Disable Alternate Vector Table  BSLIM=Not used  WDTEN=Disable  BTSWP=BOOTSWP instruction is disabled  DBCC=No Cross Connection between DAC outputs  CTXT1=Not Assigned  CTXT2=Not Assigned  SEQNUM=Not used  nSEQNUM=Not used  BOREN0=Enabled  DMTIVT=Not used  DMTCNT=2^8 (256)  DMTEN=Dead Man Timer is Disabled and can be enabled by software  ON=Not used  USERID=Not used  RESERVED1=Not used  PGL1WAY=Allow only one reconfiguration  FPLLRNG=34-68 MHz Input  FPLLICLK=FRC is input to the System PLL  FPLLMULT=PLL Multiply by 128  UPLLFSEL=USB PLL input is 24 MHz  DMTINTV=Window/Interval value is 127/128 counter value  WDTSPGM=WDT stops during Flash programming  FDMTEN=Deadman Timer is disabled  TRCEN=Trace features in the CPU are enabled  BOOTISA=Boot code and Exception code is MIPS32  FECCCON=ECC and Dynamic ECC are disabled (ECCCON bits are writable)  EXTDDRSIZE=Not used  FSLEEP=Flash is powered down when the device is in Sleep mode  DBGPER=Allow CPU access to all permission regions  EJTAGBEN=Normal EJTAG functionality  TSEQ=Not used  CSEQ=Not used
      settings: SourceProductName=MPLAB® Device Blocks for Simulink®
  Open board doc WWW : Subsystem
      settings: OpenFcn=|
      | web('www.microchip.com/www.microchip.com/en556208','-browser');
      | pause(1);
      | web('www.microchip.com/TCAD0014178791','-browser');
      mask Display: disp('Microstick Plus\nDev Board');
  PIL Profiling : MCHP_Blockset/Profiling/PIL Profiling  TIMER_Ressource=Dynamic Options  TIMER_Ressource_TXT=No constraints [Prefered]  TIMER_Ressource_Custom=[1]  TIMER_Resolution=Dynamic Options  TIMER_Resolution_TXT="Resol: 32(us)  -  MaxPer: 2.1(s)"  MCHP_TIMER_REQUEST={TIMER for PIL}{TmrCfg}20:1:1:0:[]:16777216;  MCHP_TIMER_RESULT=[3 65535 ]  MCHP_MASTERLINK=MicrostickII_ExternalMode/Microstick2 - dsPIC33EP128MC202/Microchip Master  Info="Timer 3:  Resol: 3.656359352(us)  -  Max value: 239.62(ms)"
      settings: SourceProductName=MPLAB® Device Blocks for Simulink®
  Port Info : MCHP_Blockset/System Info/Port Info  MCHP_MASTERLINK=MicrostickII_ExternalMode/Microstick2 - dsPIC33EP128MC202/Microchip Master
      settings: SourceProductName=MPLAB® Device Blocks for Simulink®
  Simulink Reset Config : MCHP_Blockset/System Configuration/Simulink Reset Config  MCHP_MASTERLINK=0
      settings: SourceProductName=MPLAB® Device Blocks for Simulink®
  Timer Info : MCHP_Blockset/System Info/Timer Info  MCHP_MASTERLINK=MicrostickII_ExternalMode/Microstick2 - dsPIC33EP128MC202/Microchip Master
      settings: SourceProductName=MPLAB® Device Blocks for Simulink®
  UART Configuration : MCHP_Blockset/BUS UART/UART Configuration  UART_REF=1  BAUD_Choice=Dynamic Options  BAUD_Choice_TXT="460800         [-0.04%]"  BAUD_Choice_IR=Dynamic Options  BAUD_Choice_IR_TXT=[]  BAUD_Custom=115200  ALT_IO=on  PIN_RX=Dynamic Options  PIN_RX_TXT=B11 / P43 / Pin[22]  PIN_TX=Dynamic Options  PIN_TX_TXT=B10 / P42 / Pin[21]  MCHP_PORT="{UART1  Rx}{U1RX}3:0:P43;{UART1  Tx}{U1TX}3:1:P42;"  MCHP_MASTERLINK=MicrostickII_ExternalMode/Microstick2 - dsPIC33EP128MC202/Microchip Master  MCHP_COM_ExtPil=on  TX_IMPLEMENTATION=Circular Buffer  TX_IMPLEMENTATION_default=Circular Buffer  TX_INT_PRIORITY=5  TX_INT_WHEN=is empty  TX_INT_WHEN_default=is empty & last char is sent  TX_CIRCULAR_SIZE=512  TX_DMA_CHANNEL="0   (Lowest Priority)"  TX_DMA_SIZE=[]  TX_TASK_PROTECTION=Delay tasks (default)  TX_INTERRUPT_PROTECTION=Do not send on conflict (default)  TX_INTERRUPT_PROTECTION_default=Do not send on conflict (default)  RX_IMPLEMENTATION=Circular Buffer  RX_IMPLEMENTATION_default=Circular Buffer  RX_INT_PRIORITY=6  RX_INT_WHEN=receive 1 character  RX_CIRCULAR_SIZE=512  DuplexMode=Full duplex (default)  PIN_RX_Inv=off  PIN_TX_Inv=off  StopBit=1 stop bit (default)  IRDA=off  FlowControl=None  PIN_CTS=Dynamic Options  PIN_CTS_TXT=B0 / P32 / Pin[4]  PIN_RTS=Dynamic Options  PIN_RTS_TXT=A4 / P20 / Pin[12]  InitSequence_chkbox=off  BAUD_Choice_InitSeq=Dynamic Options  BAUD_Choice_InitSeq_TXT="110         [+0.00%]"  BAUD_Choice_IR_InitSeq=Dynamic Options  BAUD_Choice_IR_InitSeq_TXT=0  BAUD_Custom_InitSeq=0  InitSequence='Hello World'
      settings: SourceProductName=MPLAB® Device Blocks for Simulink®
  wires:
  1Hz Blinking2/1(Out1) -> LED - Blue - RB15/1

== system MicrostickII_ExternalMode/Sin ==
  In1 : Inport
  Sin Double - Reference : Subsystem
  Sin Q15 : Subsystem
  Out1 : Outport
  Out2 : Outport  Port=2
  wires:
  In1/1 -> Sin Q15/1(In2), Sin Double - Reference/1(In1)
  Sin Q15/1(Sin_Out1) -> Out1/1
  Sin Double - Reference/1(Out1) -> Out2/1
  [Validation] -> Sin Double - Reference/Enable

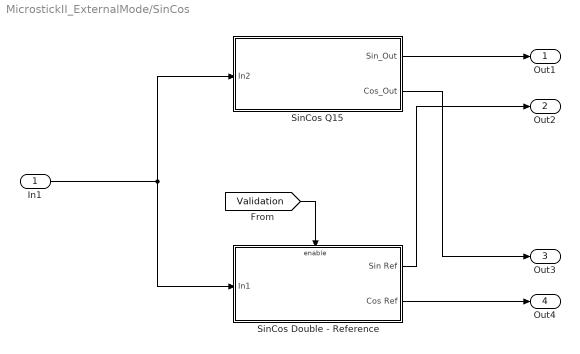
== system MicrostickII_ExternalMode/SinCos ==
  In1 : Inport
  SinCos Double - Reference : Subsystem
  SinCos Q15 : Subsystem
  Out1 : Outport
  Out2 : Outport  Port=2
  Out3 : Outport  Port=3
  Out4 : Outport  Port=4
  wires:
  In1/1 -> SinCos Q15/1(In2), SinCos Double - Reference/1(In1)
  SinCos Double - Reference/1(Sin Ref) -> Out2/1
  SinCos Double - Reference/2(Cos Ref) -> Out4/1
  SinCos Q15/2(Cos_Out) -> Out3/1
  SinCos Q15/1(Sin_Out) -> Out1/1
  [Validation] -> SinCos Double - Reference/Enable

== system MicrostickII_ExternalMode/Sqrt ==
  In1 : Inport
  " Sqrt Q15" : Subsystem  TreatAsAtomicUnit=on
  "Sqrt Double - Reference " : Subsystem  TreatAsAtomicUnit=on
  Out1 : Outport
  Out2 : Outport  Port=2
  wires:
  In1/1 -> " Sqrt Q15"/1(In1), "Sqrt Double - Reference "/1(In1)
  " Sqrt Q15"/1(Out1) -> Out1/1
  "Sqrt Double - Reference "/1(Out2) -> Out2/1
  [Validation] -> "Sqrt Double - Reference "/Enable

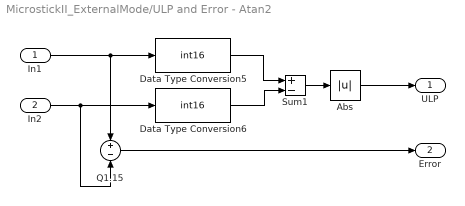
== system MicrostickII_ExternalMode/ULP and Error - Atan2 ==
  In1 : Inport
  In2 : Inport  Port=2
  Abs : Abs  SaturateOnIntegerOverflow=on
  Data Type Conversion5 : DataTypeConversion  OutDataTypeStr=int16  ConvertRealWorld=Stored Integer (SI)
  Data Type Conversion6 : DataTypeConversion  OutDataTypeStr=int16  ConvertRealWorld=Stored Integer (SI)
  Q1.15 : Sum  Inputs=+-  OutDataTypeStr=single
  Sum1 : Sum  Inputs=+-  SaturateOnIntegerOverflow=on  OutDataTypeStr=Inherit: Same as first input
  ULP : Outport
  Error : Outport  Port=2
  wires:
  Abs/1 -> ULP/1
  Q1.15/1 -> Error/1
  In1/1 -> Q1.15/1, Data Type Conversion5/1
  In2/1 -> Data Type Conversion6/1, Q1.15/2
  Sum1/1 -> Abs/1
  Data Type Conversion5/1 -> Sum1/1
  Data Type Conversion6/1 -> Sum1/2

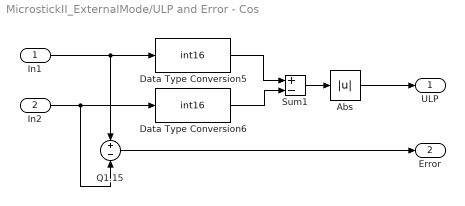
== system MicrostickII_ExternalMode/ULP and Error - Cos ==
  In1 : Inport
  In2 : Inport  Port=2
  Abs : Abs  SaturateOnIntegerOverflow=on
  Data Type Conversion5 : DataTypeConversion  OutDataTypeStr=int16  ConvertRealWorld=Stored Integer (SI)
  Data Type Conversion6 : DataTypeConversion  OutDataTypeStr=int16  ConvertRealWorld=Stored Integer (SI)
  Q1.15 : Sum  Inputs=+-  OutDataTypeStr=single
  Sum1 : Sum  Inputs=+-  SaturateOnIntegerOverflow=on  OutDataTypeStr=Inherit: Same as first input
  ULP : Outport
  Error : Outport  Port=2
  wires:
  Abs/1 -> ULP/1
  Q1.15/1 -> Error/1
  In1/1 -> Q1.15/1, Data Type Conversion5/1
  In2/1 -> Data Type Conversion6/1, Q1.15/2
  Sum1/1 -> Abs/1
  Data Type Conversion5/1 -> Sum1/1
  Data Type Conversion6/1 -> Sum1/2

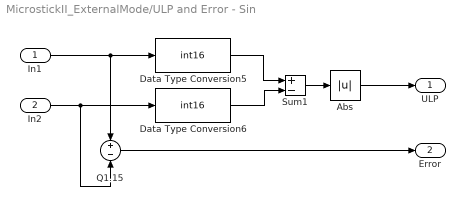
== system MicrostickII_ExternalMode/ULP and Error - Sin ==
  In1 : Inport
  In2 : Inport  Port=2
  Abs : Abs  SaturateOnIntegerOverflow=on
  Data Type Conversion5 : DataTypeConversion  OutDataTypeStr=int16  ConvertRealWorld=Stored Integer (SI)
  Data Type Conversion6 : DataTypeConversion  OutDataTypeStr=int16  ConvertRealWorld=Stored Integer (SI)
  Q1.15 : Sum  Inputs=+-  OutDataTypeStr=single
  Sum1 : Sum  Inputs=+-  SaturateOnIntegerOverflow=on  OutDataTypeStr=Inherit: Same as first input
  ULP : Outport
  Error : Outport  Port=2
  wires:
  Data Type Conversion6/1 -> Sum1/2
  Data Type Conversion5/1 -> Sum1/1
  Sum1/1 -> Abs/1
  In2/1 -> Q1.15/2, Data Type Conversion6/1
  In1/1 -> Data Type Conversion5/1, Q1.15/1
  Q1.15/1 -> Error/1
  Abs/1 -> ULP/1

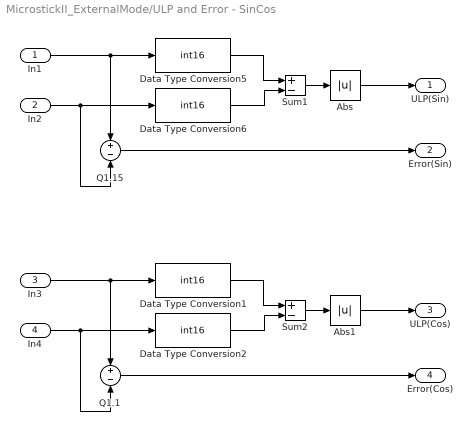
== system MicrostickII_ExternalMode/ULP and Error - SinCos ==
  In1 : Inport
  In2 : Inport  Port=2
  In3 : Inport  Port=3
  In4 : Inport  Port=4
  Abs : Abs  SaturateOnIntegerOverflow=on
  Abs1 : Abs  SaturateOnIntegerOverflow=on
  Data Type Conversion{1..2,5..6} (4 alike) : DataTypeConversion  OutDataTypeStr=int16  ConvertRealWorld=Stored Integer (SI)
  Q1.1 : Sum  Inputs=+-  OutDataTypeStr=single
  Q1.15 : Sum  Inputs=+-  OutDataTypeStr=single
  Sum1 : Sum  Inputs=+-  SaturateOnIntegerOverflow=on  OutDataTypeStr=Inherit: Same as first input
  Sum2 : Sum  Inputs=+-  SaturateOnIntegerOverflow=on  OutDataTypeStr=Inherit: Same as first input
  ULP(Sin) : Outport
  Error(Sin) : Outport  Port=2
  ULP(Cos) : Outport  Port=3
  Error(Cos) : Outport  Port=4
  wires:
  Data Type Conversion6/1 -> Sum1/2
  Data Type Conversion5/1 -> Sum1/1
  Sum1/1 -> Abs/1
  In2/1 -> Q1.15/2, Data Type Conversion6/1
  In1/1 -> Data Type Conversion5/1, Q1.15/1
  Q1.15/1 -> Error(Sin)/1
  Abs/1 -> ULP(Sin)/1
  Abs1/1 -> ULP(Cos)/1
  Q1.1/1 -> Error(Cos)/1
  In3/1 -> Q1.1/1, Data Type Conversion1/1
  In4/1 -> Data Type Conversion2/1, Q1.1/2
  Sum2/1 -> Abs1/1
  Data Type Conversion1/1 -> Sum2/1
  Data Type Conversion2/1 -> Sum2/2

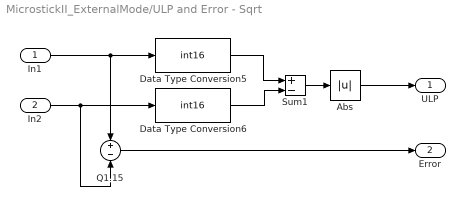
== system MicrostickII_ExternalMode/ULP and Error - Sqrt ==
  In1 : Inport
  In2 : Inport  Port=2
  Abs : Abs  SaturateOnIntegerOverflow=on
  Data Type Conversion5 : DataTypeConversion  OutDataTypeStr=int16  ConvertRealWorld=Stored Integer (SI)
  Data Type Conversion6 : DataTypeConversion  OutDataTypeStr=int16  ConvertRealWorld=Stored Integer (SI)
  Q1.15 : Sum  Inputs=+-  OutDataTypeStr=single
  Sum1 : Sum  Inputs=+-  SaturateOnIntegerOverflow=on  OutDataTypeStr=Inherit: Same as first input
  ULP : Outport
  Error : Outport  Port=2
  wires:
  Data Type Conversion6/1 -> Sum1/2
  Data Type Conversion5/1 -> Sum1/1
  Sum1/1 -> Abs/1
  In2/1 -> Q1.15/2, Data Type Conversion6/1
  In1/1 -> Data Type Conversion5/1, Q1.15/1
  Q1.15/1 -> Error/1
  Abs/1 -> ULP/1

== system MicrostickII_ExternalMode/Atan2/Atan2 Q15 ==
  In1 : Inport
  Atan2_Q1.15 : Subsystem  TreatAsAtomicUnit=on
  Demux : Demux  Outputs=2
  Out1 : Outport
  wires:
  Atan2_Q1.15/1(Out1) -> Out1/1
  Demux/1 -> Atan2_Q1.15/1(In1)
  Demux/2 -> Atan2_Q1.15/2(In2)
  In1/1 -> Demux/1

== system MicrostickII_ExternalMode/Atan2/Double Atan2 - Reference ==
  In1 : Inport
  Enable : EnablePort
  Demux : Demux  Outputs=2
  Simulink_Q1.15 : Subsystem  TreatAsAtomicUnit=on
  Simulink_Out_Q1.15 : Outport
  wires:
  Simulink_Q1.15/1(Out1) -> Simulink_Out_Q1.15/1
  In1/1 -> Demux/1
  Demux/1 -> Simulink_Q1.15/1(In1)
  Demux/2 -> Simulink_Q1.15/2(In2)

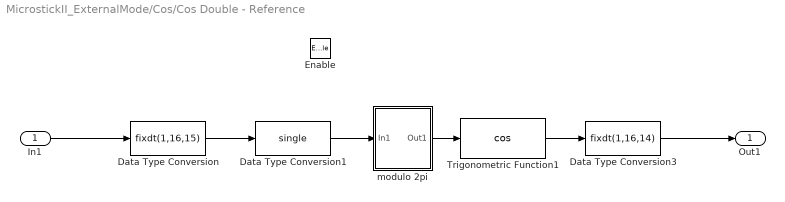
== system MicrostickII_ExternalMode/Cos/Cos Double - Reference ==
  In1 : Inport
  Enable : EnablePort
  Data Type Conversion : DataTypeConversion  OutDataTypeStr=fixdt(1,16,15)  ConvertRealWorld=Stored Integer (SI)
  Data Type Conversion1 : DataTypeConversion  OutDataTypeStr=single
  Data Type Conversion3 : DataTypeConversion  OutDataTypeStr=fixdt(1,16,14)  RndMeth=Convergent  SaturateOnIntegerOverflow=on
  Trigonometric Function1 : Trigonometry  Operator=cos  NumberOfIterations=15
  modulo 2pi : Subsystem
  Out1 : Outport
  wires:
  In1/1 -> Data Type Conversion/1
  Trigonometric Function1/1 -> Data Type Conversion3/1
  Data Type Conversion/1 -> Data Type Conversion1/1
  Data Type Conversion1/1 -> modulo 2pi/1(In1)
  modulo 2pi/1(Out1) -> Trigonometric Function1/1
  Data Type Conversion3/1 -> Out1/1

== system MicrostickII_ExternalMode/Cos/Cos Q15 ==
  In2 : Inport
  MCHP_Cos_Q1.15 : Subsystem  TreatAsAtomicUnit=on
  Cos_Out1 : Outport  OutDataTypeStr=fixdt(1,16,14)
  wires:
  In2/1 -> MCHP_Cos_Q1.15/1(In1)
  MCHP_Cos_Q1.15/1(Out1) -> Cos_Out1/1

== system MicrostickII_ExternalMode/Microstick2 - dsPIC33EP128MC202/1Hz Blinking2 ==
  Delay : Delay  DelayLength=1  InitialCondition=0  InputProcessing=Inherited  SampleTime=.5
  Logical Operator : Logic  Operator=NOT  AllPortsSameDT=off  OutDataTypeStr=boolean
  Rate Transition2 : RateTransition  Deterministic=off  OutPortSampleTime=.05
  Out1 : Outport
  wires:
  Delay/1 -> Logical Operator/1
  Logical Operator/1 -> Delay/1, Rate Transition2/1
  Rate Transition2/1 -> Out1/1

== system MicrostickII_ExternalMode/Microstick2 - dsPIC33EP128MC202/Open board doc WWW ==

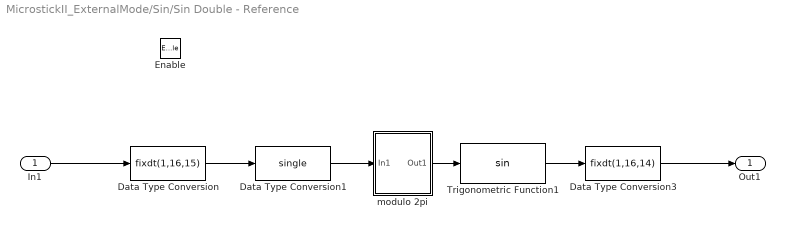
== system MicrostickII_ExternalMode/Sin/Sin Double - Reference ==
  In1 : Inport
  Enable : EnablePort
  Data Type Conversion : DataTypeConversion  OutDataTypeStr=fixdt(1,16,15)  ConvertRealWorld=Stored Integer (SI)
  Data Type Conversion1 : DataTypeConversion  OutDataTypeStr=single
  Data Type Conversion3 : DataTypeConversion  OutDataTypeStr=fixdt(1,16,14)  RndMeth=Convergent  SaturateOnIntegerOverflow=on
  Trigonometric Function1 : Trigonometry  NumberOfIterations=15
  modulo 2pi : Subsystem
  Out1 : Outport
  wires:
  Data Type Conversion3/1 -> Out1/1
  modulo 2pi/1(Out1) -> Trigonometric Function1/1
  Data Type Conversion1/1 -> modulo 2pi/1(In1)
  Data Type Conversion/1 -> Data Type Conversion1/1
  Trigonometric Function1/1 -> Data Type Conversion3/1
  In1/1 -> Data Type Conversion/1

== system MicrostickII_ExternalMode/Sin/Sin Q15 ==
  In2 : Inport
  MCHP_Sin_Q1.15 : Subsystem  TreatAsAtomicUnit=on
  Sin_Out1 : Outport  OutDataTypeStr=fixdt(1,16,14)
  wires:
  MCHP_Sin_Q1.15/1(Out1) -> Sin_Out1/1
  In2/1 -> MCHP_Sin_Q1.15/1(In1)

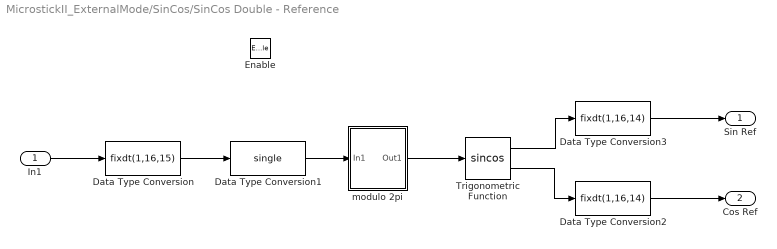
== system MicrostickII_ExternalMode/SinCos/SinCos Double - Reference ==
  In1 : Inport
  Enable : EnablePort
  Data Type Conversion : DataTypeConversion  OutDataTypeStr=fixdt(1,16,15)  ConvertRealWorld=Stored Integer (SI)
  Data Type Conversion1 : DataTypeConversion  OutDataTypeStr=single
  Data Type Conversion2 : DataTypeConversion  OutDataTypeStr=fixdt(1,16,14)  RndMeth=Convergent  SaturateOnIntegerOverflow=on
  Data Type Conversion3 : DataTypeConversion  OutDataTypeStr=fixdt(1,16,14)  RndMeth=Convergent  SaturateOnIntegerOverflow=on
  Trigonometric Function : Trigonometry  Operator=sincos
  modulo 2pi : Subsystem
  Sin Ref : Outport
  Cos Ref : Outport  Port=2
  wires:
  Data Type Conversion3/1 -> Sin Ref/1
  modulo 2pi/1(Out1) -> Trigonometric Function/1
  Data Type Conversion1/1 -> modulo 2pi/1(In1)
  Data Type Conversion/1 -> Data Type Conversion1/1
  Trigonometric Function/1 -> Data Type Conversion3/1
  In1/1 -> Data Type Conversion/1
  Data Type Conversion2/1 -> Cos Ref/1
  Trigonometric Function/2 -> Data Type Conversion2/1

== system MicrostickII_ExternalMode/SinCos/SinCos Q15 ==
  In2 : Inport
  MCHP_SinCos_Q1.15 : Subsystem  TreatAsAtomicUnit=on
  Sin_Out : Outport  OutDataTypeStr=fixdt(1,16,14)
  Cos_Out : Outport  Port=2  OutDataTypeStr=fixdt(1,16,14)
  wires:
  MCHP_SinCos_Q1.15/1(Out1) -> Sin_Out/1
  In2/1 -> MCHP_SinCos_Q1.15/1(In1)
  MCHP_SinCos_Q1.15/2(Out2) -> Cos_Out/1

== system MicrostickII_ExternalMode/Sqrt/ Sqrt Q15 ==
  In1 : Inport
  Sqrt : Sqrt  OutDataTypeStr=fixdt(1,16,15)
  Out1 : Outport
  wires:
  Sqrt/1 -> Out1/1
  In1/1 -> Sqrt/1

== system MicrostickII_ExternalMode/Sqrt/Sqrt Double - Reference  ==
  In1 : Inport
  Enable : EnablePort
  Data Type Conversion8 : DataTypeConversion  OutDataTypeStr=single
  Sqrt1 : Sqrt  OutDataTypeStr=fixdt(1,16,15)  RndMeth=Convergent
  Out2 : Outport
  wires:
  Sqrt1/1 -> Out2/1
  Data Type Conversion8/1 -> Sqrt1/1
  In1/1 -> Data Type Conversion8/1

== system MicrostickII_ExternalMode/Atan2/Atan2 Q15/Atan2_Q1.15 ==
  In1 : Inport
  In2 : Inport  Port=2
  Atan2 : Trigonometry  Operator=atan2  ApproximationMethod=CORDIC  NumberOfIterations=15  OutputSignalType=real
  Out1 : Outport
  wires:
  In1/1 -> Atan2/1
  In2/1 -> Atan2/2
  Atan2/1 -> Out1/1

== system MicrostickII_ExternalMode/Atan2/Double Atan2 - Reference/Simulink_Q1.15 ==
  In1 : Inport
  In2 : Inport  Port=2
  Data Type Conversion1 : DataTypeConversion  OutDataTypeStr=single
  Data Type Conversion3 : DataTypeConversion  OutDataTypeStr=single
  Data Type Conversion4 : DataTypeConversion  OutDataTypeStr=fixdt(1,16,13)  RndMeth=Convergent  SaturateOnIntegerOverflow=on
  Trigonometric Function1 : Trigonometry  Operator=atan2  NumberOfIterations=14  OutputSignalType=real
  Out1 : Outport
  wires:
  In2/1 -> Data Type Conversion3/1
  In1/1 -> Data Type Conversion1/1
  Data Type Conversion1/1 -> Trigonometric Function1/1
  Data Type Conversion3/1 -> Trigonometric Function1/2
  Trigonometric Function1/1 -> Data Type Conversion4/1
  Data Type Conversion4/1 -> Out1/1

== system MicrostickII_ExternalMode/Cos/Cos Double - Reference/modulo 2pi ==
  In1 : Inport
  Bias : Bias  Bias=pi
  Bias1 : Bias  Bias=-pi
  Constant2 : Constant  Value=2*pi  OutDataTypeStr=single  SampleTime=-1
  Math Function : Math  Operator=mod  SaturateOnIntegerOverflow=on
  Out1 : Outport
  wires:
  Bias1/1 -> Out1/1
  Bias/1 -> Math Function/1
  Constant2/1 -> Math Function/2
  Math Function/1 -> Bias1/1
  In1/1 -> Bias/1

== system MicrostickII_ExternalMode/Cos/Cos Q15/MCHP_Cos_Q1.15 ==
  In1 : Inport
  Cos : Trigonometry  Operator=cos  ApproximationMethod=CORDIC  NumberOfIterations=16
  Out1 : Outport
  wires:
  In1/1 -> Cos/1
  Cos/1 -> Out1/1

== system MicrostickII_ExternalMode/Sin/Sin Double - Reference/modulo 2pi ==
  In1 : Inport
  Bias : Bias  Bias=pi
  Bias1 : Bias  Bias=-pi
  Constant2 : Constant  Value=2*pi  OutDataTypeStr=single  SampleTime=-1
  Math Function : Math  Operator=mod  SaturateOnIntegerOverflow=on
  Out1 : Outport
  wires:
  In1/1 -> Bias/1
  Math Function/1 -> Bias1/1
  Constant2/1 -> Math Function/2
  Bias/1 -> Math Function/1
  Bias1/1 -> Out1/1

== system MicrostickII_ExternalMode/Sin/Sin Q15/MCHP_Sin_Q1.15 ==
  In1 : Inport
  Sin : Trigonometry  ApproximationMethod=CORDIC  NumberOfIterations=16
  Out1 : Outport
  wires:
  Sin/1 -> Out1/1
  In1/1 -> Sin/1

== system MicrostickII_ExternalMode/SinCos/SinCos Double - Reference/modulo 2pi ==
  In1 : Inport
  Bias : Bias  Bias=pi
  Bias1 : Bias  Bias=-pi
  Constant2 : Constant  Value=2*pi  OutDataTypeStr=single  SampleTime=-1
  Math Function : Math  Operator=mod  SaturateOnIntegerOverflow=on
  Out1 : Outport
  wires:
  In1/1 -> Bias/1
  Math Function/1 -> Bias1/1
  Constant2/1 -> Math Function/2
  Bias/1 -> Math Function/1
  Bias1/1 -> Out1/1

== system MicrostickII_ExternalMode/SinCos/SinCos Q15/MCHP_SinCos_Q1.15 ==
  In1 : Inport
  SinCos : Trigonometry  Operator=sincos  ApproximationMethod=CORDIC  NumberOfIterations=16
  Out1 : Outport
  Out2 : Outport  Port=2
  wires:
  SinCos/1 -> Out1/1
  In1/1 -> SinCos/1
  SinCos/2 -> Out2/1
